simulink model "Pararquanser"  (R2016a)
settings: Solver=VariableStepAuto  StartTime=0.0  StopTime=inf  RelTol=1e-3
undefined symbols (not defined in the file or in its folder): National_Instruments, PCI
libraries: sldrtlib x2, simulink x1
settings Model: Creator=luis.vasquez  LastModifiedBy=daniel.tobon

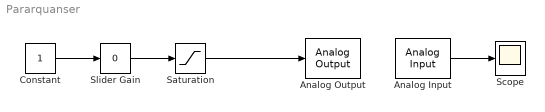
== system Pararquanser ==
  Analog Input : sldrtlib/Analog Input  SampleTime=0.1  MaxMissedTicks=10  ShowMissedTicks=off  YieldWhenWaiting=off  DrvName=National_Instruments/PCI-6221  DrvAddress=4294967295  DrvOptions=[1 0 0 0 0]  Channels=4  RangeMode=1  VoltRange=2  DataType=1
      settings: AttributesFormatString=National Instruments\nPCI-6221 [auto]
  Analog Output : sldrtlib/Analog Output  SampleTime=0.1  MaxMissedTicks=10  ShowMissedTicks=off  YieldWhenWaiting=off  DrvName=National_Instruments/PCI-6221  DrvAddress=4294967295  DrvOptions=[1 0 0 0 0]  Channels=1  RangeMode=1  VoltRange=1  InitialValue=[]  FinalValue=[]
      settings: AttributesFormatString=National Instruments\nPCI-6221 [auto]
  Constant : Constant
  Saturation : Saturate  UpperLimit=5  LowerLimit=0
  Scope : Scope
  Slider Gain : simulink/Math Operations/Slider Gain  low=0  gain=0  high=5
  wires:
  Constant/1 -> Slider Gain/1
  Saturation/1 -> Analog Output/1
  Analog Input/1 -> Scope/1
  Slider Gain/1 -> Saturation/1
